simulink model "c12_ConsensusDelaysModel1"  (R2020b)
settings: Solver=VariableStepAuto  StartTime=0.0  StopTime=t_end  MaxStep=0.01  MinStep=0.001  RelTol=1e-3
values from neighbouring files (symbols this model uses):
  L = Hbar'*W*Hbar    [c12_MultipleDelaysLMI.m]    (also in c14_bipartite_MWconsensus_animation.m = [A12+A13 -A12        -A13           Z                   Z   )
  tau = 1    [c12_delayAdaptive.m]
  x0 = 5    [c12_delayAdaptive.m]    (also in c14_bipartite_MWconsensus_animation.m = [x0;r/norm(r)]; c15_closed_model.m = 5*rand(15,1); c15_open_model.m = 5*rand(15,1))
settings Model: Creator=HoangMinh  LastModifiedBy=trinh

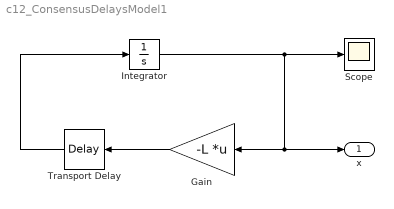
== system c12_ConsensusDelaysModel1 ==
  Gain : Gain  Gain=-L  Multiplication=Matrix(K*u) (u vector)
  Integrator : Integrator  InitialCondition=x0
  Scope : Scope
  Transport Delay : TransportDelay  DelayTime=tau
  x : Outport  SignalName=x
  wires:
  Gain/1 -> Transport Delay/1
  Transport Delay/1 -> Integrator/1
  Integrator/1 -> Scope/1, Gain/1, x/1
